simulink model "Project_ACS_Microgrid_Dynamics_Simulation_And_Test_2018a"  (R2018a)
settings: Solver=VariableStepAuto  StartTime=0.0  StopTime=2  MaxStep=1e-4  RelTol=1e-2
undefined symbols (not defined in the file): powergui, rt
libraries: powerlib x25, powerlib_meascontrol x16, simulink x7
(part 2 of 2)

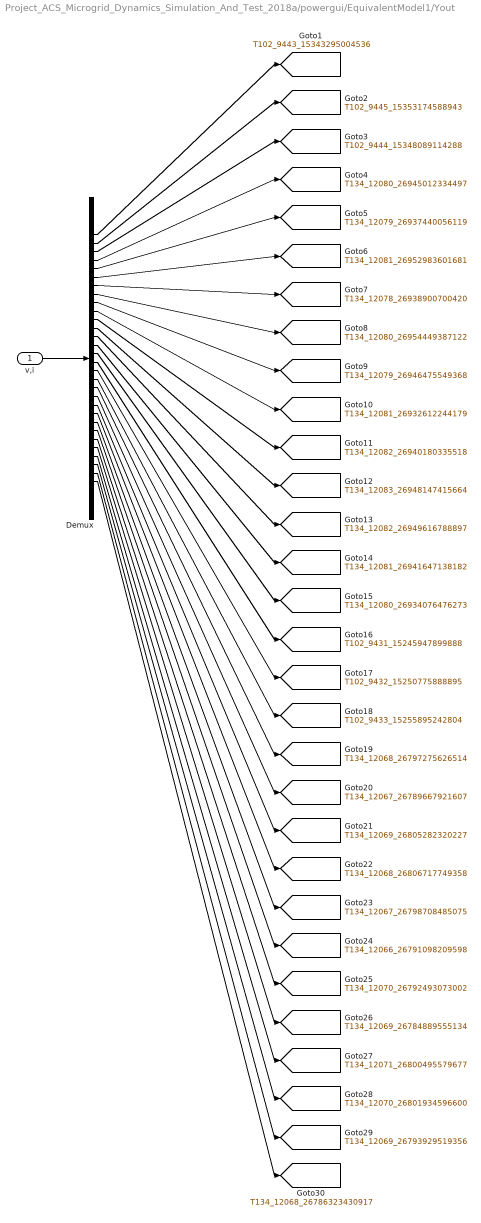
== system Project_ACS_Microgrid_Dynamics_Simulation_And_Test_2018a/powergui/EquivalentModel1/Yout ==
  v,i : Inport
  Demux : Demux  Outputs=[1 1 1 1 1 1 1 1 1 1 1 1 1 1 1 1 1 1 1 1 1 1 1 1 1 1 1 1 1 1]
  tag scope: T102_9431_15245947899888=global, T102_9432_15250775888895=global, T102_9433_15255895242804=global, T102_9443_15343295004536=global, T102_9444_15348089114288=global, T102_9445_15353174588943=global, T134_12066_26791098209598=global, T134_12067_26789667921607=global, T134_12067_26798708485075=global, T134_12068_26786323430917=global, T134_12068_26797275626514=global, T134_12068_26806717749358=global, T134_12069_26784889555134=global, T134_12069_26793929519356=global, T134_12069_26805282320227=global, T134_12070_26792493073002=global, T134_12070_26801934596600=global, T134_12071_26800495579677=global, T134_12078_26938900700420=global, T134_12079_26937440056119=global, T134_12079_26946475549368=global, T134_12080_26934076476273=global, T134_12080_26945012334497=global, T134_12080_26954449387122=global, T134_12081_26932612244179=global, T134_12081_26941647138182=global, T134_12081_26952983601681=global, T134_12082_26940180335518=global, T134_12082_26949616788897=global, T134_12083_26948147415664=global
  wires:
  v,i/1 -> Demux/1
  Demux/1 -> [T102_9443_15343295004536]
  Demux/2 -> [T102_9445_15353174588943]
  Demux/3 -> [T102_9444_15348089114288]
  Demux/4 -> [T134_12080_26945012334497]
  Demux/5 -> [T134_12079_26937440056119]
  Demux/6 -> [T134_12081_26952983601681]
  Demux/7 -> [T134_12078_26938900700420]
  Demux/8 -> [T134_12080_26954449387122]
  Demux/9 -> [T134_12079_26946475549368]
  Demux/10 -> [T134_12081_26932612244179]
  Demux/11 -> [T134_12082_26940180335518]
  Demux/12 -> [T134_12083_26948147415664]
  Demux/13 -> [T134_12082_26949616788897]
  Demux/14 -> [T134_12081_26941647138182]
  Demux/15 -> [T134_12080_26934076476273]
  Demux/16 -> [T102_9431_15245947899888]
  Demux/17 -> [T102_9432_15250775888895]
  Demux/18 -> [T102_9433_15255895242804]
  Demux/19 -> [T134_12068_26797275626514]
  Demux/20 -> [T134_12067_26789667921607]
  Demux/21 -> [T134_12069_26805282320227]
  Demux/22 -> [T134_12068_26806717749358]
  Demux/23 -> [T134_12067_26798708485075]
  Demux/24 -> [T134_12066_26791098209598]
  Demux/25 -> [T134_12070_26792493073002]
  Demux/26 -> [T134_12069_26784889555134]
  Demux/27 -> [T134_12071_26800495579677]
  Demux/28 -> [T134_12070_26801934596600]
  Demux/29 -> [T134_12069_26793929519356]
  Demux/30 -> [T134_12068_26786323430917]
